simulink model "nopid"  (R2019a)
settings: Solver=VariableStepAuto  StartTime=0.0  StopTime=10  MaxStep=1e-3  RelTol=1e-3
libraries: fl_lib x6, nesl_utility x3, ee_lib x3
settings Model: Creator=ooloncolluphid  LastModifiedBy=Oolon Colluphid

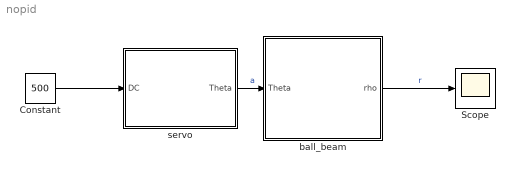
== system nopid ==
  Constant : Constant  Value=500
  Scope : Scope
  ball_beam : Subsystem
  servo : Subsystem
  wires:
  servo/1(Theta) -> ball_beam/1(Theta)  "a"
  ball_beam/1(rho) -> Scope/1  "r"
  Constant/1 -> servo/1(DC)

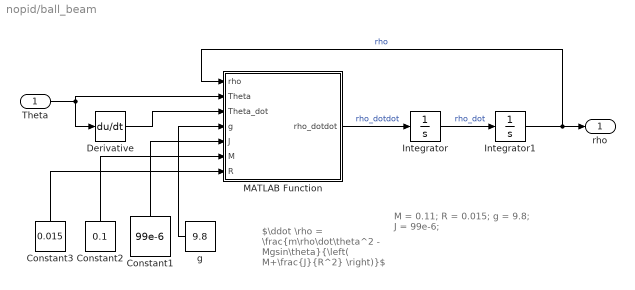
== system nopid/ball_beam ==
  note: M = 0.11;
      | R = 0.015;
      | g = 9.8;
      | J = 99e-6;
  note: $\ddot \rho = \frac{m\rho\dot\theta^2 - Mgsin\theta}{\left( M+\frac{J}{R^2} \right)}$
  Theta : Inport
  Constant1 : Constant  Value=99e-6
  Constant2 : Constant  Value=0.1
  Constant3 : Constant  Value=0.015
  Derivative : Derivative
  Integrator : Integrator
  Integrator1 : Integrator
  MATLAB Function : MATLAB Function  TreatAsAtomicUnit=on
  g : Constant  Value=9.8
  rho : Outport
  wires:
  g/1 -> MATLAB Function/4(g)
  Theta/1 -> Derivative/1, MATLAB Function/2(Theta)
  Constant2/1 -> MATLAB Function/6(M)
  Integrator1/1 -> rho/1, MATLAB Function/1(rho)  "rho"
  MATLAB Function/1(rho_dotdot) -> Integrator/1  "rho_dotdot"
  Constant3/1 -> MATLAB Function/7(R)
  Constant1/1 -> MATLAB Function/5(J)
  Derivative/1 -> MATLAB Function/3(Theta_dot)
  Integrator/1 -> Integrator1/1  "rho_dot"

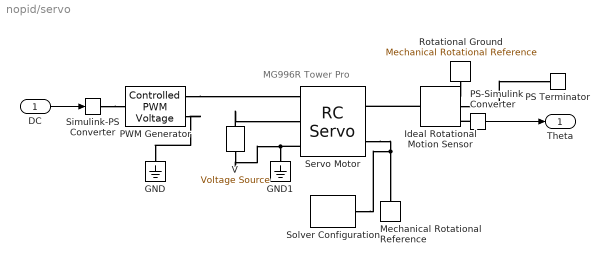
== system nopid/servo ==
  note: MG996R Tower Pro
  DC : Inport
  GND : fl_lib/Electrical/Electrical Elements/Electrical Reference
  GND1 : fl_lib/Electrical/Electrical Elements/Electrical Reference
  Ideal Rotational Motion Sensor : fl_lib/Mechanical/Mechanical Sensors/Ideal Rotational Motion Sensor  offset=0 deg
  Mechanical Rotational Reference : fl_lib/Mechanical/Rotational Elements/Mechanical Rotational Reference
  PS Terminator : fl_lib/Physical Signals/Sinks/PS Terminator
      settings: SourceProductName=Simscape
  PS-Simulink Converter : nesl_utility/PS-Simulink Converter  PhysicalDomain=network_engine_domain  SubClassName=ps_output  LeftPortType=input  RightPortType=output  PseudoPeriodic=off  Frequencies=[]  Unit=1  AffineConversion=off
  PWM Generator : ee_lib/Integrated Circuits/Controlled PWM Voltage  F=50 Hz  TD=0 s  pulse_width_offset=0 s  pulse_min=0 s  Vmin=0 V  Vmax=5 V  Vm=4.8 V  pwm_or_av=1  event_type=1  sample_time=1e-6 s  u_min=0  u_max=65536
      settings: SourceProductName=Simscape Electrical
  Rotational Ground : fl_lib/Mechanical/Rotational Elements/Mechanical Rotational Reference
  Servo Motor : ee_lib/Electromechanical/Brushed Motors/RC Servo  stall_torque=9.4 kg*cm  time_60=0.17 s  nominal_voltage=4.8 V  rotational_range=[-60 +60] deg  pulse_width_range=[1, 2] ms  threshold=3 V  R_s=18 kOhm  resolution=0.1 deg  angle_meas_error=0 deg  backdrive_torque=0.5 kg*cm  ratio=320  inertia=0.01 g*cm^2  endstop_angles=[-65, 65] deg  endstop_stiffness=1e6 N*m/rad  endstop_damping=0.01 N*m/(rad/s)  enable_faults=0  fault_action=1  fault_type=1  enable_temporal_fault=0  t_fault=1 s  enable_behavioral_fault=0  max_permissible_current=1 A  t_fail_on_current=1 s  angle_specify=on  angle_priority=High  angle=0 deg  angle_nominal_specify=off  angle_nominal_unit=deg  angle_nominal_value=1  w_specify=off  w_priority=High  w=0 deg/s  w_nominal_specify=off  w_nominal_unit=deg/s  w_nominal_value=1  torque_specify=off  torque_priority=High  torque=0 N*m  torque_nominal_specify=off  torque_nominal_unit=N*m  torque_nominal_value=1  pulse_width_specify=off  pulse_width_priority=None  pulse_width=1.5 ms  i_specify=off  i_priority=None  i=0 A  i_nominal_specify=off  i_nominal_unit=A  i_nominal_value=1  i_s_specify=off  i_s_priority=None  i_s=0 A  i_s_nominal_specify=off  i_s_nominal_unit=A  i_s_nominal_value=1  motor_torque_specify=off  motor_torque_priority=None  motor_torque=0 N*m  motor_torque_nominal_specify=off  motor_torque_nominal_unit=N*m  motor_torque_nominal_value=1  power_dissipated_specify=off  power_dissipated_priority=None  power_dissipated=0 W  power_dissipated_nominal_specify=off  power_dissipated_nominal_unit=W  power_dissipated_nominal_value=1  angle_demand_specify=off  angle_demand_priority=None  angle_demand=90 deg  angle_demand_nominal_specify=off  angle_demand_nominal_unit=deg  angle_demand_nominal_value=1  faulted_specify=off  faulted_priority=None  faulted=0  faulted_nominal_specify=off  faulted_nominal_unit=1  faulted_nominal_value=1
      settings: SourceProductName=Simscape Electrical  SourceProductBaseCode=PS
  Simulink-PS Converter : nesl_utility/Simulink-PS Converter  PhysicalDomain=network_engine_domain  SubClassName=ps_input  LeftPortType=input  RightPortType=output  PseudoPeriodic=off  Frequencies=[]  NoiseDistribution=none  NoiseParameters=[]  Unit=1  AffineConversion=off  FilteringAndDerivatives=provide  SimscapeFilterOrder=1  InputFilterTimeConstant=0.001  UdotUserProvided=0
  Solver Configuration : nesl_utility/Solver Configuration  PhysicalDomain=network_engine_domain  SubClassName=solver  LeftPortType=input  RightPortType=generic  Tones=[]  Harmonics=[]  SimulateNoise=off  Profile=off  UseLocalSampling=off  EnableSwitchedLinearOptims=on  FrequencyDomain=off  UseCCode=off  RelTol=0.001  AbsTol=1e-06  MinStep=1e-09  ToWorkspace=off  RevertToSquareIcSolve=off  NumHomotopyIterations=100  PhasorMode=off  PhasorModeNumHarmonics=1  DoDC=off  ResidualTolerance=1e-09  UseLocalSolver=off  LocalSolverChoice=NE_BACKWARD_EULER_ADVANCER  LocalSolverSampleTime=0.001  DoFixedCost=off  MaxNonlinIter=3  MaxModeIter=2  LinearAlgebra=auto  EquationFormulation=NE_TIME_EF  DelaysMemoryBudget=1024  AutomaticFiltering=on  FilteringTimeConstant=0.001  PartitionStorageMethod=AS_NEEDED  PartitionMemoryBudget=1024  PartitionMethod=ROBUST
  V : ee_lib/Sources/Voltage Source  dc_voltage=5 V  ac_voltage=0 V  ac_shift=0 rad  ac_frequency=60 Hz  noise_mode=0  PSD=0 V^2/Hz  repeatability=1  auto_seed=3499211588  user_seed=0  sample_time=1e-3 s  i_specify=off  i_priority=None  i=0 A  i_nominal_specify=off  i_nominal_unit=A  i_nominal_value=1  v_specify=off  v_priority=None  v=0 V  v_nominal_specify=off  v_nominal_unit=V  v_nominal_value=1
      settings: SourceProductName=Simscape Electrical
  Theta : Outport
  wires:
  PS-Simulink Converter/1 -> Theta/1
  DC/1 -> Simulink-PS Converter/1
  connections:
  Ideal Rotational Motion Sensor/LConn1 -- Servo Motor/RConn1
  GND1/LConn1 -- Servo Motor/LConn3 -- V/RConn1
  V/LConn1 -- Servo Motor/LConn2
  PWM Generator/RConn2 -- GND/LConn1
  Rotational Ground/LConn1 -- Ideal Rotational Motion Sensor/RConn1
  PWM Generator/RConn1 -- Servo Motor/LConn1
  PS-Simulink Converter/LConn1 -- Ideal Rotational Motion Sensor/RConn3
  Solver Configuration/RConn1 -- Servo Motor/RConn2 -- Mechanical Rotational Reference/LConn1
  Ideal Rotational Motion Sensor/RConn2 -- PS Terminator/LConn1
  Simulink-PS Converter/RConn1 -- PWM Generator/LConn1

== matlab function nopid/ball_beam/MATLAB Function ==
  data: rho input; rho_dotdot output; Theta input; Theta_dot input; g input; J input; M input; R input
function rho_dotdot = fcn(rho, Theta, Theta_dot, g, J, M, R)

rho_dotdot = ((M*g*sin(Theta))) - (M*rho*Theta_dot^2) / ...
        ((J/(R^2)) + M);
